simulink library "GenericTarget"  (R2025b)
settings: Solver=VariableStepAuto  StartTime=0.0  StopTime=10.0  RelTol=1e-3
undefined symbols (not defined in the file or in its folder): GT_CheckUniqueParameterValue, strlength
libraries: simulink x4, $bdroot x2, etargetslib x1
(part 3 of 3)

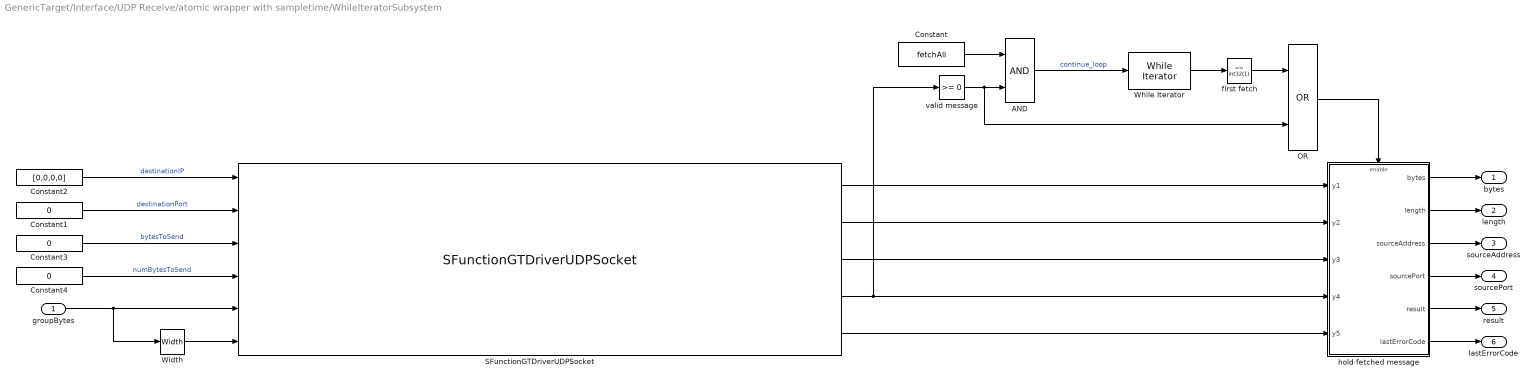
== system GenericTarget/Interface/UDP Receive/atomic wrapper with sampletime/WhileIteratorSubsystem ==
  groupBytes : Inport
  AND : Logic  AllPortsSameDT=off  OutDataTypeStr=boolean
  Constant : Constant  Value=fetchAll
  Constant1 : Constant  Value=0  OutDataTypeStr=uint16
  Constant2 : Constant  Value=[0,0,0,0]  OutDataTypeStr=uint8
  Constant3 : Constant  Value=0  OutDataTypeStr=uint8
  Constant4 : Constant  Value=0  OutDataTypeStr=int32
  OR : Logic  Operator=OR  AllPortsSameDT=off  OutDataTypeStr=boolean
  SFunctionGTDriverUDPSocket : S-Function  FunctionName=SFunctionGTDriverUDPSocket  Parameters=SParameter1, SParameter2, SParameter3, SParameter4, SParameter5, SParameter6, SParameter7, SParameter8, SParameter9, SParameter10, SParameter11, SParameter12, SampleTime  SFunctionDeploymentMode=off  EnableBusSupport=off  mask(Legacy Function){SFunctionSpec=void GT_DriverUDPSocketStep(int32 p1, uint8 p11, int32 p12, uint8 y1[p12], uint8 y2[4], uint16 y3[1], int32 y4[1], int32 y5[1], uint8 u1[4], uint16 u2, uint8 u3[], int32 u4, uint8 u5[], uint32 u6), SParameter1=int32(reshape(localPort, [1 1])), SParameter2=[uint8(deviceName),uint8(0)], SParameter3=uint32(numel(deviceName)), SParameter4=int32(reshape(socketPriority, [1 1])), SParameter5=uint8(reshape(allowBroadcast, [1 1])), SParameter6=uint8(reshape(allowZeroLengthMessage, [1 1])), SParameter7=uint8(reshape(multicastAll, [1 1])), SParameter8=uint8(reshape(multicastLoop, [1 1])), SParameter9=uint8(reshape(multicastTTL, [1 1])), SParameter10=uint8(reshape(multicastInterfaceAddress, [1 4])), SParameter11=uint8(0), SParameter12=int32(reshape(rxBufferSize, [1 1])), SampleTime=-1, ShowSpec=off}
      mask prompts: SParameter1 "P1:"; SParameter2 "P2:"; SParameter3 "P3:"; SParameter4 "P4:"; SParameter5 "P5:"; SParameter6 "P6:"; SParameter7 "P7:"; SParameter8 "P8:"; SParameter9 "P9:"; SParameter10 "P10:"; SParameter11 "P11:"; SParameter12 "P12:"; SampleTime "Sample time (-1 for inherited):"; ShowSpec "Display function specification"
      mask help:
      | This block allows you to call the legacy functions specified by the following Legacy Code Tool definition:
      | def.SFunctionName = 'SFunctionGTDriverUDPSocket';
      | def.OutputFcnSpec = 'void GT_DriverUDPSocketStep(int32 p1, uint8 p11, int32 p12, uint8 y1[p12], uint8 y2[4], uint16 y3[1], int32 y4[1], int32 y5[1], uint8 u1[4], uint16 u2, uint8 u3[], int32 u4, uint8 u5[], uint32 u6)';
      | def.StartFcnSpec = 'void GT_DriverUDPSocketInitialize(int32 p1, uint8 p2[], uint32 p3, int32 p4, uint8 p5, uint8 p6, uint8 p7, uint8 p8, uint8 p9, uint8 p10[4])';
      | def.TerminateFcnSpec = 'void GT_DriverUDPSocketTerminate(int32 p1)';
      | def.HeaderFiles = {'GT_DriverUDPSocket.hpp'};
      | def.SourceFiles = {'GT_DriverUDPSocket.cpp', 'GT_DriverImplementationDetails.cpp'};
      | def.SampleTime = 'parameterized';
      | def.Options.useTlcWithAccel = false;
      | def.Options.language = 'C++';
      mask Help: <p>This block was generated automatically by the Legacy Code Tool. For detailed help on this tool, call<a href="matlab:legacy_code('help')"> legacy_code('help')</a>.</p>
      mask Callback ShowSpec:
      | if strcmp(get_param(gcbh, 'ShowSpec'), 'on')
      |   set_param(gcbh, 'MaskDisplay', sprintf('fprintf(''%s'');', get_param(gcbh, 'SFunctionSpec')));
      | else
      |   set_param(gcbh, 'MaskDisplay', sprintf('fprintf(''%s'');', get_param(gcbh, 'FunctionName')));
      | end
      mask Display: fprintf('SFunctionGTDriverUDPSocket');
  While Iterator : WhileIterator  MaxIters=-1  WhileBlockType=do-while  ShowIterationPort=on
  Width : Width  DataType=uint32
  first fetch : simulink/Logic and Bit Operations/Compare To Constant  relop===  const=int32(1)  OutDataTypeStr=boolean
  hold fetched message : Subsystem  TreatAsAtomicUnit=on
  valid message : simulink/Logic and Bit Operations/Compare To Zero  relop=>=  OutDataTypeStr=boolean
  bytes : Outport
  length : Outport  Port=2
  sourceAddress : Outport  Port=3
  sourcePort : Outport  Port=4
  result : Outport  Port=5
  lastErrorCode : Outport  Port=6
  wires:
  SFunctionGTDriverUDPSocket/2 -> hold fetched message/2(y2)
  SFunctionGTDriverUDPSocket/3 -> hold fetched message/3(y3)
  SFunctionGTDriverUDPSocket/1 -> hold fetched message/1(y1)
  SFunctionGTDriverUDPSocket/4 -> hold fetched message/4(y4), valid message/1
  groupBytes/1 -> SFunctionGTDriverUDPSocket/5, Width/1
  SFunctionGTDriverUDPSocket/5 -> hold fetched message/5(y5)
  valid message/1 -> OR/2, AND/2
  AND/1 -> While Iterator/1  "continue_loop"
  hold fetched message/6(lastErrorCode) -> lastErrorCode/1
  hold fetched message/5(result) -> result/1
  hold fetched message/3(sourceAddress) -> sourceAddress/1
  hold fetched message/4(sourcePort) -> sourcePort/1
  hold fetched message/1(bytes) -> bytes/1
  While Iterator/1 -> first fetch/1
  first fetch/1 -> OR/1
  OR/1 -> hold fetched message/Enable
  Constant/1 -> AND/1
  Width/1 -> SFunctionGTDriverUDPSocket/6
  Constant2/1 -> SFunctionGTDriverUDPSocket/1  "destinationIP"
  Constant1/1 -> SFunctionGTDriverUDPSocket/2  "destinationPort"
  Constant3/1 -> SFunctionGTDriverUDPSocket/3  "bytesToSend"
  Constant4/1 -> SFunctionGTDriverUDPSocket/4  "numBytesToSend"
  hold fetched message/2(length) -> length/1

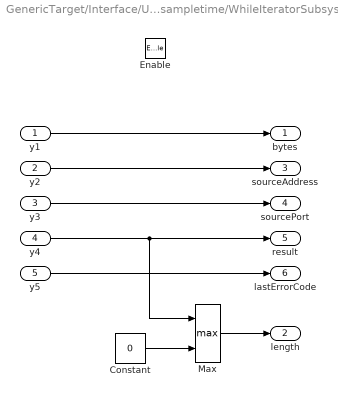
== system GenericTarget/Interface/UDP Receive/atomic wrapper with sampletime/WhileIteratorSubsystem/hold fetched message ==
  y1 : Inport
  y2 : Inport  Port=2
  y3 : Inport  Port=3
  y4 : Inport  Port=4
  y5 : Inport  Port=5
  Enable : EnablePort
  Constant : Constant  Value=0  OutDataTypeStr=int32
  Max : MinMax  Function=max  Inputs=2
  bytes : Outport
  length : Outport  Port=2
  sourceAddress : Outport  Port=3
  sourcePort : Outport  Port=4
  result : Outport  Port=5
  lastErrorCode : Outport  Port=6
  wires:
  y1/1 -> bytes/1
  y3/1 -> sourcePort/1
  y2/1 -> sourceAddress/1
  y4/1 -> Max/1, result/1
  y5/1 -> lastErrorCode/1
  Max/1 -> length/1
  Constant/1 -> Max/2
